simulink model "Autonomous_SF"  (Simulink 7.7)
settings: Solver=ode4  StartTime=0.0  StopTime=inf  FixedStep=sample_time  RelTol=1e-3
InitFcn:
  | sample_time=0.02;
  | DeltaT = sample_time;
  | H0 = -0.3;
  | Kl = 1;
undefined symbols (not defined in the file or in its folder): DiscIntNeverNeededParam
libraries: simulink x6, utility x1, dspadpt3 x1
(part 2 of 2)

== system Autonomous_SF/Vicon_Data/Raw Quad Pose from Vicon3/Process Vicon Raw Data/Flip_pi1/Flip_0_to_2pi/Flip_2pi ==
  Angle : Inport
  Bias : Bias  Bias=-2*pi
  Constant : Constant  Value=2*pi
  Data Type Duplicate : DataTypeDuplicate
  Modulo : Math  Operator=mod  SaturateOnIntegerOverflow=on
  Sign1 : Signum
  Switch : Switch
  Angle_Flip : Outport
  wires:
  Switch/1 -> Data Type Duplicate/2, Angle_Flip/1
  Bias/1 -> Switch/3
  Sign1/1 -> Switch/2
  Modulo/1 -> Switch/1, Bias/1
  Constant/1 -> Modulo/2
  Angle/1 -> Data Type Duplicate/1, Sign1/1, Modulo/1

== system Autonomous_SF/Vicon_Data/Raw Quad Pose from Vicon3/Process Vicon Raw Data1/Flip_pi1/Flip_0_to_2pi/Flip_2pi ==
  Angle : Inport
  Bias : Bias  Bias=-2*pi
  Constant : Constant  Value=2*pi
  Data Type Duplicate : DataTypeDuplicate
  Modulo : Math  Operator=mod  SaturateOnIntegerOverflow=on
  Sign1 : Signum
  Switch : Switch
  Angle_Flip : Outport
  wires:
  Angle/1 -> Modulo/1, Sign1/1, Data Type Duplicate/1
  Constant/1 -> Modulo/2
  Modulo/1 -> Bias/1, Switch/1
  Sign1/1 -> Switch/2
  Bias/1 -> Switch/3
  Switch/1 -> Angle_Flip/1, Data Type Duplicate/2

== system Autonomous_SF/Vicon_Data/Raw Quad Pose from Vicon3/Process Vicon Raw Data2/Flip_pi1/Flip_0_to_2pi/Flip_2pi ==
  Angle : Inport
  Bias : Bias  Bias=-2*pi
  Constant : Constant  Value=2*pi
  Data Type Duplicate : DataTypeDuplicate
  Modulo : Math  Operator=mod  SaturateOnIntegerOverflow=on
  Sign1 : Signum
  Switch : Switch
  Angle_Flip : Outport
  wires:
  Switch/1 -> Data Type Duplicate/2, Angle_Flip/1
  Bias/1 -> Switch/3
  Sign1/1 -> Switch/2
  Modulo/1 -> Switch/1, Bias/1
  Constant/1 -> Modulo/2
  Angle/1 -> Data Type Duplicate/1, Sign1/1, Modulo/1

== matlab function Yaw Controller/MATLAB Function ==
  data: u input double; y output double
function y = fcn(u)
%#codegen
y = u;
if y > pi    
    y = y - 2*pi;
elseif y < -pi
        y = y + 2*pi;
end

== stateflow chart Trajectory Logic/UAV SF ==
  state Landing
    state Decsending
      en:PosDesired = Pos;
      du:PosDesired[2] = (0 - PosDesired[2])*1*DeltaT + PosDesired[2] ;
    state CutThrottle
      du:HoverThrottle = (-0.95 - HoverThrottle)*2*DeltaT + HoverThrottle ;
    (default) -> Decsending
    Decsending -> CutThrottle : [Pos[2] > -0.15]
  state Airborne
    state TakeOff
      du:HoverThrottle = (H0 - HoverThrottle)*2*DeltaT + HoverThrottle ;
    state Perching
    state Hover
    state Trajectory
      du:
      VelCmd[0] = VelCmd(-RC[2]);
      VelCmd[1] = VelCmd(RC[1]);
      PosDesired[0] = PosDesired[0] + DeltaT*VelCmd[0];
      PosDesired[1] = PosDesired[1] + DeltaT*VelCmd[1];
    (default) -> TakeOff : {PosDesired = Pos;  PosDesired[2] = -1;}
    TakeOff -> Hover : after(5,sec)
        | {PosDesired = Pos;}
    Hover -> Trajectory : [RC[5] > 0]
    Trajectory -> Hover : [RC[5] < 0]
        | {PosDesired = Pos;}
  state y=VelCmd(u) [function]
  (default) -> Landing
  Airborne -> Landing : [RC[6] < -0.5]
  Landing -> Airborne : [RC[6] > 0.5]
  data: u function_input double; y function_output double; PosDesired output double size=4; HoverThrottle output double size=1; Mode output uint8 size=3; RC input double size=8; Pos input double size=4; PerchPos input double size=4; DeltaT parameter double size=1; H0 parameter double size=1; Kl parameter double size=1; VelCmd local double size=2 =0
